simulink model "Tipo4_v4"  (R2018b)
(part 2 of 6)

  Three-Phase Series RLC Branch : powerlib/Elements/Three-Phase Series RLC Branch  LConnTagsString=A|B|C  RConnTagsString=A|B|C  BranchType=RL  Resistance=(500e3^2/2.2e9)/10  Inductance=(500e3^2/2.2e9)/377  Capacitance=0  Measurements=None
  Three-Phase Series RLC Branch1 : powerlib/Elements/Three-Phase Series RLC Branch  LConnTagsString=A|B|C  RConnTagsString=A|B|C  BranchType=RL  Resistance=0.191366666666667*18  Inductance=0.002053833333333*18  Capacitance=0  Measurements=None
  Three-Phase Series RLC Branch2 : powerlib/Elements/Three-Phase Series RLC Branch  LConnTagsString=A|B|C  RConnTagsString=A|B|C  BranchType=RL  Resistance=0.214533333333333*1.37  Inductance=0.001806666666667*1.37  Capacitance=0  Measurements=None
  Wind Turbine Type 4 : Subsystem  LoadFcn=%find_system(gcs,'FollowLinks', 'on', 'LookUnderMasks', 'all');  mask(Wind Turbine: Model 7){Nb_wt=110, ShowParameters=Generator data for 1 wind turbine, nom=[2e6/0.9 730 60], Reactances=[ 1.305, 0.296, 0.252, 0.474,  0.243,  0.18 ], Time_constants=[  4.49  0.0681  0.0513  ], Resistance=0.006, mec=[0.62 0.01 1], init=[ 0  0  0  0  0  0  0  0  1 ], Vnom=575, Imax_grid_conv=1.1, RL_grid=[ 0.15 0.15/50], C_var_filter1=150e3, Vdc_nom=1100, C_DClink1=90000e-6, L_R_Boost=[0.0012     5e-3], Pmec1=2e6, wind_speed_CpMax=11, wind0=11, DisplayTurbChar=off, H_WT=4.32, Ksh=0.3, D_mutual=1.5, w_wt0=1, torque0=1, Kdc=[1.1   27.5], Ki_var_reg=0.05, Ki_volt_reg=2, Kgrid_side_cur_reg=[1  50], Kspeed=[5 1], Kboost_cur_reg=[0.025 100], Kp_pitch=15, Kcompensation=[1.5  6], Kfield=[10  20], pitch_max=27, pitch_rate=10, Ts=Ts}
      mask prompts: Nb_wt "Number of wind turbines:"; ShowParameters "Display:"; nom "Nom. power, L-L volt. and freq.: [Pn (VA), Vn (Vrms), fn (Hz)]"; Reactances "Reactances [Xd Xd' Xd'' Xq Xq'' Xl] (p.u.):"; Time_constants "Time constants [Tdo' Tdo'' Tq''] (s):"; Resistance "Resistance Rs (p.u.):"; mec "Inertia constant, friction factor, and pairs of poles: [ H(s)  F(p.u.)  p ]"; init "Initial conditions: [dw(%) th(deg) ia,ib,ic(pu) pha,phb,phc(deg) Vf(pu)]:"; Vnom "Grid-side converter nominal AC voltage (V):"; Imax_grid_conv "Grid-side converter maximum AC current (pu based on generator power and converter nominal AC voltage):"; RL_grid "Grid-side coupling inductor [ L(pu) R(pu),pu based on generator power and converter nominal AC voltage] :"; C_var_filter1 "Line filter capacitor (Q=50) (var):"; Vdc_nom "Nominal DC bus voltage (V)"; C_DClink1 "DC bus capacitor (F):"; L_R_Boost "Boost converter inductance [L(H) R(ohm)]:"; Pmec1 "Nominal mechanical output power (W):"; wind_speed_CpMax "Wind speed at nominal speed and at Cp max (must be between 6 m/s and 30 m/s) (m/s):"; wind0 "Initial wind speed (m/s):"; DisplayTurbChar "Display wind turbine power characteristics:"; H_WT "Wind turbine inertia constant H (s):"; Ksh "Shaft spring constant refer to high-speed shaft (pu of nominal mechanical torque/rad):"; D_mutual "Shaft mutual damping (pu of nominal mechanical torque/pu dw):"; w_wt0 "Turbine initial speed (pu of nominal speed):"; torque0 "Initial output torque (pu of nominal mechanical torque):"; Kdc "DC bus voltage regulator gains [Kp Ki]:"; Ki_var_reg "Grid-side converter var regulator gain [ Ki]:"; Ki_volt_reg "Grid-side converter voltage regulator gain [ Ki]:"; Kgrid_side_cur_reg "Grid-side converter current regulator gains [Kp Ki]:"; Kspeed "Speed regulator gains [Kp Ki]:"; Kboost_cur_reg "Boost inductor current regulator gains [Kp Ki]:"; Kp_pitch "Pitch controller gain [Kp]:"; Kcompensation "Pitch compensation gains [Kp Ki]:"; Kfield "Field excitation gains [Kp Ki]:"; pitch_max "Maximum pitch angle (deg):"; pitch_rate "Maximum rate of change of pitch angle (deg/s)"; Ts "Sample time (s):"
      mask help: This block implements a model of a variable speed pitch controlled wind turbine using a synchronous generator.
      mask init:
      | %Generator data
      | Pnom=nom(1)*Nb_wt;
      | Vnom_gen=nom(2);
      | Fnom=nom(3);
      | Xd=Reactances(1);
      | Xd1=Reactances(2);
      | Xd2=Reactances(3);
      | Xq=Reactances(4);
      | Xq2=Reactances(5);
      | Xl=Reactances(6);
      | Tdo1=Time_constants(1);
      | Tdo2=Time_constants(2);
      | Tq2=Time_constants(3);
      | H=mec(1);
      | F=mec(2);
      | p=mec(3);
      | 
      | % Converters data
      | L_RL=RL_grid(1);
      | R_RL=RL_grid(2);
      | L_Boost=L_R_Boost(1)/Nb_wt;
      | R_Boost=L_R_Boost(2)/Nb_wt;
      | Q_filter=50;
      | C_DClink=C_DClink1*Nb_wt;
      | C_var_filter=C_var_filter1*Nb_wt;
      | 
      | % Controller data
      | Freq_filter=10000;   %Hz
      | Zeta_filter=0.707;
      | Kp_dc=Kdc(1);
      | Ki_dc=Kdc(2);
      | Kp_grid_side_cur_reg=Kgrid_side_cur_reg(1);
      | Ki_grid_side_cur_reg=Kgrid_side_cur_reg(2);
      | Kp_speed=Kspeed(1);
      | Ki_speed=Kspeed(2);
      | Kp_boost_cur_reg=Kboost_cur_reg(1);
      | Ki_boost_cur_reg=Kboost_cur_reg(2);
      | Kp_compensation=Kcompensation(1);
      | Ki_compensation=Kcompensation(2);
      | Kp_field=Kfield(1);
      | Ki_field=Kfield(2);
      | Mod_index_max=1.1;
      | T_speed=5;      %Speed reference time constant (s)
      | Iq_ref_limit_time_constant=0.3; %(s)
      | Current_reg_output_limit=1.1;   %(pu)
      | Var_reg_output_hi_limit=1.1;    %(pu)
      | Var_reg_output_low_limit=0.9;   %(pu)
      | Pitch_time_constant=0.01;       %(s)
      | Vf_limit=10;    %Field voltage limit (pu)
      | Flux_meas_time_constant=1*(1/Fnom); %(s)
      | Freq_sawtooth=2000; %Hz, Boost converter
      | Freq_PWM=3000; %Hz, Inverter
      | Ts_snub=50e-6;  %Sample time to compute snubber resistance
      | 
      | 
      | % Turbine data
      | Pmec=Pmec1*Nb_wt;
      | c1 = 0.6450;
      | c2 = 116;
      | c3 = .4;
      | c4 = 5;
      | c5 = 21;
      | c6 = .00912;  % Set Pmin in stall condition (does not vary with wind_speed_Pmax)
      | c7 = .08;
      | c8 = .035;
      | theta=0;
      | CpMax=.5;
      | lambda_CpMax=9.9495;
      | 
      | c1_c8=[c1 c2 c3 c4 c5 c6 c7 c8];
      |   
      | 
      | %   Cp = c1*(c6*lambda + (-c4 - c3*(2.5 + theta) + c2*(1/(lambda + ...
      | %   c7*(2.5 + theta)) - c8/(1 + (2.5 + theta)^3)))/exp(c5*(1/(lambda + ...
      | %   c7*(2.5 + theta)) - c8/(1 + (2.5 + theta)^3))))
      | 
      | 
      |         %%%%%%%%%%%%%%%%%%%%%%%%%%%%%%%%%%%%%%%%%%%%%%%%%%%%%%%%%%%%%%%%%%%%%%%%%%%
      |         % Operation at Cp max
      |         %%%%%%%%%%%%%%%%%%%%%%%%%%%%%%%%%%%%%%%%%%%%%%%%%%%%%%%%%%%%%%%%%%%%%%%%%%%
      |         
      |         rated_omegar=1;
      |         omegar = rated_omegar;
      |         
      |         % Enforce boundaries on wind speed
      |         % A warning could be displayed
      |         if wind_speed_CpMax < 6
      |             wind_speed_CpMax=6;
      |             disp('Warning: Wind speed at nominal speed and at Cp max has been set to 6 m/s')
      |         end
      |         if wind_speed_CpMax > 30
      |             wind_speed_CpMax=30;
      |             disp('Warning: Wind speed at nominal speed and at Cp max has been set to 30 m/s')
      |         end
      | 
      |         K1=lambda_CpMax/omegar*wind_speed_CpMax;
      |         
      |         % Calculation of K2 needed to get P equal to the requested value at
      |         % Cp max for the requested wind speed
      |         
      |         Prated=Pmec;
      |         P_rated_omegar_theta_zero=0.75;
      |         
      |         K2 = P_rated_omegar_theta_zero*Prated/(wind_speed_CpMax^3*CpMax);
      |         
      |         K1_K2=[K1 K2];
      |         
      |         %%%%%%%%%%%%%%%%%%%%%%%%%%%%%%%%%%%%%%%%%%%%%%%%%%%%%%%%%%%%%%%%%%%%%%%%%%%
      |         % End of calculation for operation at Cp max
      |         %%%%%%%%%%%%%%%%%%%%%%%%%%%%%%%%%%%%%%%%%%%%%%%%%%%%%%%%%%%%%%%%%%%%%%%%%%%
      |         
      | 
      | %%%%%%%%%%%%%%%%%%%%%%%%%%%%%%%%%%%%%%%%%%%%%%%%%%%%%%%%%%%%%%%%%%%%%%%%%%%
      | % Plot turbine characteristics
      | %%%%%%%%%%%%%%%%%%%%%%%%%%%%%%%%%%%%%%%%%%%%%%%%%%%%%%%%%%%%%%%%%%%%%%%%%%% 
      | 
      | DisplayTurbChar=get_param(gcb,'DisplayTurbChar');
      | if strcmp(DisplayTurbChar,'on')
      |     vect_theta = 0:2:30;
      |     
      |     vect_lambda = 1:0.2:30;
      |     
      |     clear Cp;
      |     
      |     for i=1:length(vect_theta)
      |      for j=1:length(vect_lambda)
      |                 Cp(i,j) = c1*(c6*vect_lambda(j) + (-c4 - c3*(2.5 + vect_theta(i)) + c2*(1/(vect_lambda(j) + ...
      |                 c7*(2.5 + vect_theta(i))) - c8/(1 + (2.5 + vect_theta(i))^3)))/exp(c5*(1/(vect_lambda(j) + ...
      |                 c7*(2.5 + vect_theta(i))) - c8/(1 + (2.5 + vect_theta(i))^3))));
      |      end
      |     end
      | 
      |     figure(1);
      |     clf;
      |     hold on;
      | 
      |     plot(vect_lambda, Cp);
      |     axis([0, 25, 0, .6]);
      |     title('Wind Turbine Cp Characteristic (pitch angle increases by step of 2 deg.)');
      |     ylabel('Cp');
      |     set(gca,'ytick',[0 .1 .2 .3 .4 .5 .6]);
      |     xlabel('Lambda');
      |     grid on;
      |     text(10.1,0.51,'Pitch angle 0 degree');
      | 
      |     hold off
      |     
      |     % Plot of the wind turbine mechanical power output (pu) lambda and Cp
      |     % characteristics against wind speed (m/s) for a range of theta.
      |     
      |     wind_speed_range = [1,.2,30];
      |     vect_wind_speed = 1:0.2:30;
      |     
      |     clear lambda;
      |     clear Cp;
      |     clear P;
      | 
      |     for i=1:length(vect_theta)
      |         for j=1:length(vect_wind_speed)
      |             lambda(i,j) = K1*omegar/vect_wind_speed(j);
      |             Cp(i,j) = c1*(c6*lambda(i,j) + (-c4 - c3*(2.5 + vect_theta(i)) + c2*(1/(lambda(i,j) + ...
      |             c7*(2.5 + vect_theta(i))) - c8/(1 + (2.5 + vect_theta(i))^3)))/exp(c5*(1/(lambda(i,j) + ...
      |             c7*(2.5 + vect_theta(i))) - c8/(1 + (2.5 + vect_theta(i))^3))));
      |             P(i,j) = K2/Prated*vect_wind_speed(j)^3*Cp(i,j);
      |         end
      |     end
      |     
      |     
      |     figure(2);
      |     clf;
      |     hold on
      |     
      |     subplot(3,1,1);
      |     plot(vect_wind_speed, P);
      |     axis([0, 35, 0, 1.5]);
      |     title('Wind Turbine Characteristics (w = 1 pu, pitch angle increases by step of 2 deg.)');
      |     ylabel('P (pu)');
      |     set(gca,'ytick',0:.5:4);
      |     grid on;
      |     
      |     subplot(3,1,2);
      |     plot(vect_wind_speed, lambda);
      |     axis([0, 35, 0, 20]);
      |     ylabel('Lambda');
      |     grid on;
      |     
      |     subplot(3,1,3)
      |     plot(vect_wind_speed, Cp);
      |     axis([0, 35, 0, .6]);
      |     xlabel('Wind Speed (m/s)');
      |     ylabel('Cp');
      |     set(gca,'ytick',[0 .1 .2 .3 .4 .5 .6]);
      |     grid on;
      | 
      |     hold off
      |     set_param(gcb,'DisplayTurbChar','off')
      |     
      | end
      mask TypeOptions ShowParameters: Generator data for 1 wind turbine | Converters data for 1 wind turbine | Turbine data for 1 wind turbine | Drive train data for 1 wind turbine | Control parameters for 1 wind turbine
      mask Callback ShowParameters:
      | BlockName=getfullname(gcb);
      | %
      | Param_Show=get_param(BlockName,'ShowParameters');
      | Param_DisplayTurbChar=get_param(BlockName,'DisplayTurbChar');
      | 
      | p_mask{3}='off';p_mask{4}='off';p_mask{5}='off';
      | p_mask{6}='off';p_mask{7}='off';p_mask{8}='off';p_mask{9}='off';
      | p_mask{10}='off';p_mask{11}='off';p_mask{12}='off';p_mask{13}='off';
      | p_mask{14}='off';p_mask{15}='off';p_mask{16}='off';p_mask{17}='off';
      | p_mask{18}='off';p_mask{19}='off';p_mask{20}='off';p_mask{21}='off';
      | p_mask{22}='off';p_mask{23}='off';p_mask{24}='off';p_mask{25}='off';
      | p_mask{26}='off';p_mask{27}='off';p_mask{28}='off';p_mask{29}='off';
      | p_mask{30}='off';p_mask{31}='off';p_mask{32}='off';p_mask{33}='off';
      | p_mask{34}='off';p_mask{35}='off';
      | 
      | switch Param_Show
      | 	case 'Generator data for 1 wind turbine'
      | 		p_mask{3}='on';p_mask{4}='on';p_mask{5}='on';
      |         p_mask{6}='on';p_mask{7}='on';p_mask{8}='on';
      |     case 'Converters data for 1 wind turbine'
      | 		p_mask{9}='on';p_mask{10}='on';p_mask{11}='on';
      |         p_mask{12}='on';p_mask{13}='on';p_mask{14}='on';p_mask{15}='on';
      | 	case 'Turbine data for 1 wind turbine'
      | 		p_mask{16}='on';p_mask{17}='on';p_mask{18}='on';p_mask{19}='on';
      |     case 'Drive train data for 1 wind turbine'
      |         p_mask{20}='on';p_mask{21}='on';p_mask{22}='on';p_mask{23}='on';
      |         p_mask{24}='on';
      |     case 'Control parameters for 1 wind turbine'
      |         p_mask{25}='on';p_mask{26}='on';p_mask{27}='on';
      |         p_mask{28}='on';p_mask{29}='on';p_mask{30}='on';p_mask{31}='on';
      |         p_mask{32}='on';p_mask{33}='on';p_mask{34}='on';p_mask{35}='on';
      | end
      | 
      | ParVisible={'on','on',p_mask{3},p_mask{4},p_mask{5},p_mask{6},...
      |     p_mask{7},p_mask{8},p_mask{9},p_mask{10},p_mask{11},p_mask{12},...
      |     p_mask{13},p_mask{14},p_mask{15},p_mask{16},p_mask{17},p_mask{18},...
      |     p_mask{19},p_mask{20},p_mask{21},p_mask{22},p_mask{23},p_mask{24},...
      |     p_mask{25},p_mask{26},p_mask{27},p_mask{28},p_mask{29},p_mask{30},...
      |     p_mask{31},p_mask{32},p_mask{33},p_mask{34},p_mask{35},'on'};
      | %
      | set_param(BlockName,'MaskVisibilities',ParVisible);
      | set_param(BlockName,'DisplayTurbChar',Param_DisplayTurbChar);
      mask Display: disp(' ');
  powergui : powerlib/powergui  SimulationMode=Discrete  SampleTime=Ts  frequency=60  Iterations=50  frequencyindice=60  Pbase=100e6  ErrMax=1e-4  UnitsV=kV  UnitsW=MW  buscounter=0  FunctionMessages=off  echomessages=off  EnableUseOfTLC=off  CurrentSourceSwitches=off  DisableSnubberDevices=off  DisableRonSwitches=off  DisableVfSwitches=off  DisplayEquations=off  SolverType=Tustin/Backward Euler (TBE)  Interpol=off  ExternalGateDelay=off  methode=off  Ts=100  x0status=blocks  SPID=off  SwTol=0  HookPort=off  RestoreLinks=warning  ResistiveCurrentMeasurement=off  Frange=[0:0.1:90]  Ylog=off  Xlog=off  ShowGrid=off  save=on  variable=ZData  structure=Vabc_Iabc  ZoomFFT=on  StartTime=0.0  cycles=1  DisplayStyle=1  fundamental=60  FreqAxis=off  MaxFrequency=1000  frequencyindicesteady=1  RmsSteady=1  display=off
  wires:
  Terminal Remoto/1 -> MW3/1
  MW1/1 -> [V_Local]
  [P50] -> Subsystem9/1(In1)
  [P80] -> Subsystem2/1(In1)
  [P90] -> Subsystem4/1(In1)
  [P10] -> Subsystem12/1(In1)
  [P70] -> Subsystem1/1(In1)
  [P60] -> Subsystem5/1(In1)
  [P100] -> Subsystem3/1(In1)
  MW2/1 -> [I_Local]
  MW3/1 -> [V_Remoto]
  MW4/1 -> [I_Remoto]
  Terminal Remoto/2 -> MW4/1
  Compare To Constant6/1 -> [P60]
  Compare To Constant3/1 -> [P30]
  Constant1/1 -> Compare To Constant6/1, Compare To Constant7/1, Compare To Constant8/1, Compare To Constant3/1, Compare To Constant9/1, Compare To Constant10/1, Compare To Constant5/1, Compare To Constant4/1, Compare To Constant2/1, Compare To Constant1/1, Compare To Constant/1
  Compare To Constant1/1 -> [P10]
  Compare To Constant2/1 -> [P20]
  Compare To Constant8/1 -> [P80]
  Compare To Constant7/1 -> [P70]
  Compare To Constant9/1 -> [P90]
  Compare To Constant5/1 -> [P50]
  Compare To Constant/1 -> [P0]
  Compare To Constant10/1 -> [P100]
  Compare To Constant4/1 -> [P40]
  MW5/1 -> Demux1/1
  [P_pu] -> Mux1/1
  Mux1/1 -> MW5/1
  [I_Remoto] -> Demux7/1, Scope1/2, Demux3/1, Sequence Analyzer1/1, Scope2/1
  [V_Remoto] -> Demux6/1, Scope1/1, Demux2/1, Sequence Analyzer/1
  [V_Local] -> Demux8/1, Scope3/1, Demux4/1, Sequence Analyzer2/1
  Demux1/2 -> Mux2/2  "Q (Mvar)"
  Demux1/1 -> Mux2/1  "P (MW)"
  [Q_pu] -> Mux1/2
  Mux2/1 -> Scope5/1
  Constant4/1 -> Wind Turbine Type 4/2(Qref_pu)
  Constant/1 -> Wind Turbine Type 4/1("Wind (m/s) ")
  [P0] -> Subsystem11/1(In1)
  Sequence Analyzer/2 -> Mux3/2
  Sequence Analyzer/1 -> Mux3/1
  Mux3/1 -> Scope6/1
  Mux4/1 -> Scope7/1
  Sequence Analyzer1/1 -> Mux4/1
  Sequence Analyzer1/2 -> Mux4/2
  Sequence Analyzer3/1 -> Mux6/1
  Mux5/1 -> Scope8/1
  Mux6/1 -> Scope9/1
  Sequence Analyzer2/1 -> Mux5/1
  Sequence Analyzer2/2 -> Mux5/2
  Sequence Analyzer3/2 -> Mux6/2
  Demux2/1 -> Fourier/1  "P (MW)"
  Demux3/1 -> Fourier1/1  "P (MW)"
  Fourier/1 -> Scope16/1, Divide/1
  Fourier1/1 -> Scope17/1, Divide/2
  Fourier/2 -> Scope16/2, Subtract/1
  Fourier1/2 -> Scope17/2, Subtract/2
  Demux4/1 -> Fourier2/1  "P (MW)"
  Fourier3/1 -> Scope19/1, Divide1/2
  Fourier2/1 -> Scope18/1, Divide1/1
  Demux5/1 -> Fourier3/1  "P (MW)"
  Fourier2/2 -> Scope18/2, Subtract1/1
  Fourier3/2 -> Scope19/2, Subtract1/2
  Bus Selector/3 -> [P_pu]  "<P_pu>"
  Bus Selector/4 -> [Q_pu]  "<Q_pu>"
  Bus Selector/1 -> [Vdc]  "<Vdc_V>"
  Bus Selector/2 -> [wr]  "<wr_pu>"
  [P30] -> Subsystem7/1(In1)
  [P20] -> Subsystem6/1(In1)
  [P40] -> Subsystem8/1(In1)
  [I_Local] -> Scope3/2, Demux9/1, Demux5/1, Sequence Analyzer3/1, Scope4/1
  Demux6/1 -> Scope10/1  "P (MW)"
  Demux7/1 -> Scope10/2, Scope11/1  "P (MW)"
  Demux8/1 -> Scope13/1  "P (MW)"
  Demux9/1 -> Scope13/2, Scope12/1  "P (MW)"
  Polar to Cartesian/1 -> Display/1
  Polar to Cartesian/2 -> Display1/1
  Divide/1 -> Display4/1, Scope14/1, Polar to Cartesian/1
  Subtract/1 -> Display5/1, Scope14/2, Polar to Cartesian/2
  Polar to Cartesian1/1 -> Display2/1
  Polar to Cartesian1/2 -> Display3/1
  Divide1/1 -> Display6/1, Scope15/1, Polar to Cartesian1/1
  Subtract1/1 -> Display7/1, Scope15/2, Polar to Cartesian1/2
  Wind Turbine Type 4/1(m) -> Bus Selector/1
  Terminal Local/1 -> MW1/1
  Terminal Local/2 -> MW2/1
  connections:
  Distributed Parameters Line4/RConn3 -- Distributed Parameters Line5/LConn3 -- Subsystem9/RConn3
  Distributed Parameters Line/LConn3 -- Subsystem11/RConn3 -- Terminal Remoto/RConn3
  Distributed Parameters Line/LConn2 -- Subsystem11/RConn2 -- Terminal Remoto/RConn2
  Subsystem3/RConn2 -- Terminal Local/RConn2 -- Distributed Parameters Line9/RConn2
  Distributed Parameters Line9/LConn1 -- Subsystem4/RConn1 -- Distributed Parameters Line8/RConn1
  Distributed Parameters Line7/RConn2 -- Subsystem2/RConn2 -- Distributed Parameters Line8/LConn2
  Distributed Parameters Line9/LConn3 -- Subsystem4/RConn3 -- Distributed Parameters Line8/RConn3
  Distributed Parameters Line6/LConn1 -- Subsystem5/RConn1 -- Distributed Parameters Line5/RConn1
  Distributed Parameters Line5/LConn1 -- Subsystem9/RConn1 -- Distributed Parameters Line4/RConn1
  Distributed Parameters Line2/LConn1 -- Subsystem6/RConn1 -- Distributed Parameters Line1/RConn1
  Distributed Parameters Line9/LConn2 -- Subsystem4/RConn2 -- Distributed Parameters Line8/RConn2
  Subsystem3/RConn3 -- Terminal Local/RConn3 -- Distributed Parameters Line9/RConn3
  Distributed Parameters Line2/RConn3 -- Subsystem7/RConn3 -- Distributed Parameters Line3/LConn3
  Subsystem3/RConn1 -- Terminal Local/RConn1 -- Distributed Parameters Line9/RConn1
  Distributed Parameters Line6/LConn2 -- Subsystem5/RConn2 -- Distributed Parameters Line5/RConn2
  Distributed Parameters Line2/RConn1 -- Subsystem7/RConn1 -- Distributed Parameters Line3/LConn1
  Distributed Parameters Line7/LConn3 -- Subsystem1/RConn3 -- Distributed Parameters Line6/RConn3
  Distributed Parameters Line2/LConn3 -- Subsystem6/RConn3 -- Distributed Parameters Line1/RConn3
  Distributed Parameters Line6/LConn3 -- Subsystem5/RConn3 -- Distributed Parameters Line5/RConn3
  Distributed Parameters Line2/RConn2 -- Subsystem7/RConn2 -- Distributed Parameters Line3/LConn2
  Distributed Parameters Line5/LConn2 -- Subsystem9/RConn2 -- Distributed Parameters Line4/RConn2
  Distributed Parameters Line1/LConn2 -- Subsystem12/RConn2 -- Distributed Parameters Line/RConn2
  Distributed Parameters Line/LConn1 -- Subsystem11/RConn1 -- Terminal Remoto/RConn1
  Distributed Parameters Line7/LConn1 -- Subsystem1/RConn1 -- Distributed Parameters Line6/RConn1
  Distributed Parameters Line1/LConn1 -- Subsystem12/RConn1 -- Distributed Parameters Line/RConn1
  Distributed Parameters Line7/RConn3 -- Subsystem2/RConn3 -- Distributed Parameters Line8/LConn3
  Distributed Parameters Line2/LConn2 -- Subsystem6/RConn2 -- Distributed Parameters Line1/RConn2
  Distributed Parameters Line1/LConn3 -- Subsystem12/RConn3 -- Distributed Parameters Line/RConn3
  Distributed Parameters Line4/LConn3 -- Subsystem8/RConn3 -- Distributed Parameters Line3/RConn3
  Distributed Parameters Line4/LConn1 -- Subsystem8/RConn1 -- Distributed Parameters Line3/RConn1
  Distributed Parameters Line7/LConn2 -- Subsystem1/RConn2 -- Distributed Parameters Line6/RConn2
  Distributed Parameters Line4/LConn2 -- Subsystem8/RConn2 -- Distributed Parameters Line3/RConn2
  Distributed Parameters Line7/RConn1 -- Subsystem2/RConn1 -- Distributed Parameters Line8/LConn1
  Three-Phase Series RLC Branch2/LConn3 -- "138 kV/34,5 kV "/RConn3
  Three-Phase Series RLC Branch/LConn2 -- 500 kV/RConn2
  Three-Phase Series RLC Branch/LConn3 -- 500 kV/RConn3
  Three-Phase Series RLC Branch2/LConn1 -- "138 kV/34,5 kV "/RConn1
  Three-Phase Series RLC Branch2/RConn1 -- 34,5 kV/0,575 kV/LConn1
  Three-Phase Series RLC Branch/LConn1 -- 500 kV/RConn1
  Three-Phase Series RLC Branch1/RConn2 -- "138 kV/34,5 kV "/LConn2
  Three-Phase Series RLC Branch2/LConn2 -- "138 kV/34,5 kV "/RConn2
  Three-Phase Series RLC Branch1/LConn2 -- "500 kV/138 kV "/RConn2
  Three-Phase Series RLC Branch1/LConn1 -- "500 kV/138 kV "/RConn1
  Three-Phase Series RLC Branch/RConn2 -- Terminal Remoto/LConn2
  Terminal Remoto/LConn3 -- Three-Phase Series RLC Branch/RConn3
  Three-Phase Series RLC Branch1/RConn1 -- "138 kV/34,5 kV "/LConn1
  Three-Phase Series RLC Branch2/RConn3 -- 34,5 kV/0,575 kV/LConn3
  Three-Phase Series RLC Branch1/LConn3 -- "500 kV/138 kV "/RConn3
  Three-Phase Series RLC Branch2/RConn2 -- 34,5 kV/0,575 kV/LConn2
  Three-Phase Series RLC Branch1/RConn3 -- "138 kV/34,5 kV "/LConn3
  Terminal Remoto/LConn1 -- Three-Phase Series RLC Branch/RConn1
  Ground/LConn1 -- 500 kV/LConn1
  Wind Turbine Type 4/LConn2 -- 34,5 kV/0,575 kV/RConn2
  Wind Turbine Type 4/LConn1 -- 34,5 kV/0,575 kV/RConn1
  Wind Turbine Type 4/LConn3 -- 34,5 kV/0,575 kV/RConn3
  Terminal Local/LConn3 -- "500 kV/138 kV "/LConn3
  "500 kV/138 kV "/LConn2 -- Terminal Local/LConn2
  "500 kV/138 kV "/LConn1 -- Terminal Local/LConn1
